simulink model "taskGUIModel"  (R2015b)
settings: Solver=FixedStepDiscrete  StartTime=0.0  StopTime=inf  FixedStep=0.001  RelTol=1e-3
StartFcn:
  | localAddEventListener
settings Model: Creator=shenoylab  LastModifiedBy=shenoylab
settings SolverCC: EnableConcurrentExecution=on
settings DataIOCC: LimitDataPoints=off  SaveFormat=Array  SaveOutput=off  SignalLogging=off  DSMLogging=off  VisualizeSimOutput=off  SaveTime=off
settings OptimizationCC: BlockReduction=off  OptimizeBlockIOStorage=off  BufferReuse=off  GlobalBufferReuse=off  ExpressionFolding=off  LocalBlockOutputs=off
settings DebuggingCC: SaveWithDisabledLinksMsg=none  InheritedTsInSrcMsg=none
settings HardwareCC: ProdBitPerPointer=32  ProdLargestAtomicFloat=None  ProdWordSize=32  ProdLongLongMode=on  ProdHWDeviceType=Generic->32-bit x86 compatible
settings ModelReferenceCC: ModelReferenceNumInstancesAllowed=Single  PropagateVarSize=During execution
settings RTWCC: RTWCompilerOptimization=on
settings CodeAppCC: MaxIdLength=100
settings GRTTargetCC: GeneratePreprocessorConditionals=Disable all
settings ConfigComp: CovModelRefEnable=Off

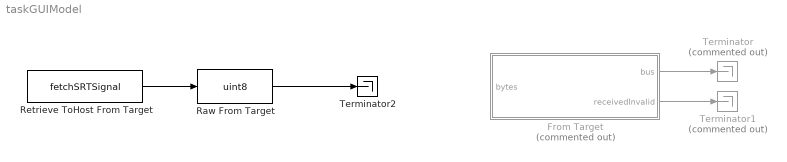
== system taskGUIModel ==
  From Target : MATLAB Function  Commented=on  TreatAsAtomicUnit=on  mask(BusSerialize: deserialize block){busType=Bus: ToHostBus}
      mask prompts: busType "Bus Type"
      mask help: Select the bus type below to deserialize into.
      mask init:
      | % BusSerialize.maskDeserializeBlockUpdate(gcb)
      | % commenting this out so that i can add a try catch block around
      | % deserialize manually
  Raw From Target : DataTypeConversion  OutDataTypeStr=uint8
  Retrieve ToHost From Target : M-S-Function  FunctionName=fetchSRTSignal  Parameters=signalIdStart,signalIdStop  mask(Get Real-Time Signal from Target){signalLabel='ToHost', signalIdStart=0, signalIdStop=0}
      mask prompts: signalLabel "Signal Label"
      mask help:
      | This block will poll the current Simulink Real-Time Target for the value of the signal with the indicated name.
      |
      | In order to make a signal visible, you can check "Signal name must resolve to a Simulink signal object" on the line properties, and then create a Simulink.Signal object by the same name in the base workspace, set signal.CoderInfo.StorageClass = 'ExportedGlobal'. Alternatively, you can change the storage class to ExportedGlobal on the Code Generation tab.
      |
      | Under the hood, this block uses tg.getsignalidsfromlabel and tg.getsignal to retrieve all elements of the vector signal, which will be output as a vector of doubles.
      mask init:
      | [signalIdStart, signalIdStop] = initFetchSRTSignal(gcb, signalLabel);
  Terminator : Terminator  Commented=on
  Terminator1 : Terminator  Commented=on
  Terminator2 : Terminator
  wires:
  From Target/1(bus) -> Terminator/1
  Retrieve ToHost From Target/1 -> Raw From Target/1
  Raw From Target/1 -> Terminator2/1
  From Target/2(receivedInvalid) -> Terminator1/1

== matlab function taskGUIModel/From Target ==
  data: bytes input; bus output Bus: ToHostBus size=1; receivedInvalid output uint8 size=1
function [bus, receivedInvalid] = deserializeWithMemory(bytes)

    % cache input so we only deserialize when input changes
    persistent pBytes;
    if isempty(pBytes)
        pBytes = bytes;
        inChanged = uint8(1);
    elseif ~isequal(pBytes, bytes)
        pBytes = bytes;
        inChanged = uint8(1);
    else
        inChanged = uint8(0);
    end
    
    persistent pInvalid;
    if isempty(pInvalid)
        pInvalid = uint8(0);
    end

    % external cached output
    persistent pBusOut;
    if isempty(pBusOut)
        pBusOut = initializeBus_ToHostBus();
    end

    % handle deserialization if changed
    if inChanged
        try
            [tempBus, valid] = deserializeBus_ToHostBus(bytes);
        catch
            valid = uint8(0);
        end
        if valid
            pBusOut = tempBus;
            pInvalid = uint8(0);
        else
            pInvalid = uint8(1);
        end
    end
         
    bus = pBusOut;
    receivedInvalid = pInvalid;
end
